simulink model "sampleModel1919"  (R2023a)
settings: Solver=VariableStepAuto  StartTime=0.0  StopTime=10.0  RelTol=1e-3
libraries: hdlsllib x6, simulink x1
settings Model: Creator=user1  LastModifiedBy=user1

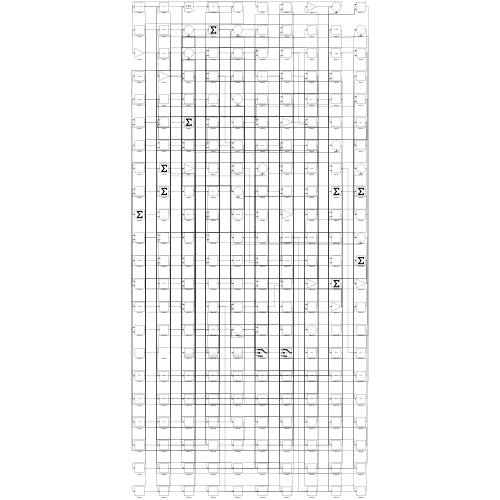
[thumbnail: Simulink's stored preview of the top-level diagram]
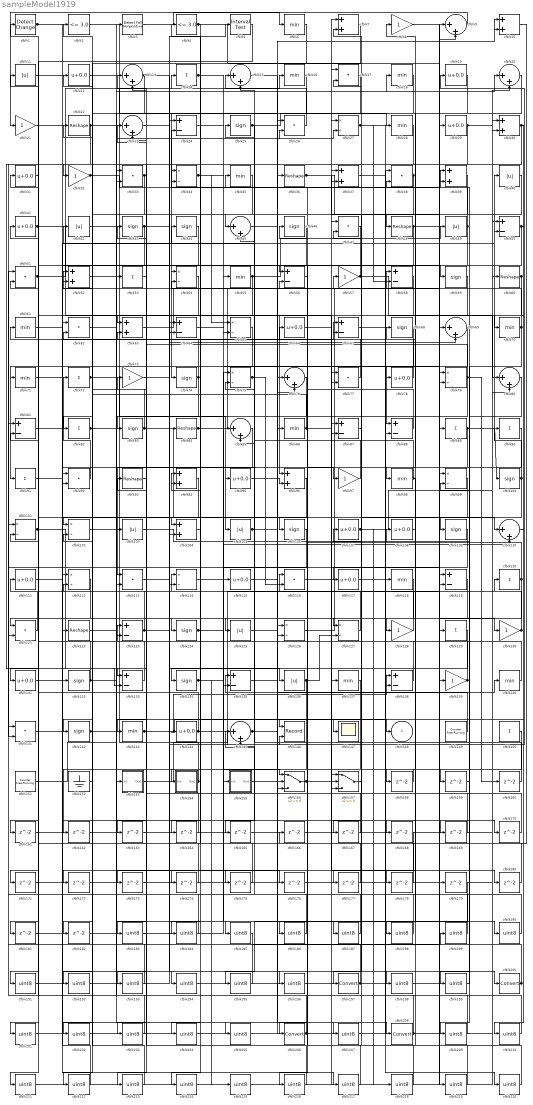
== system sampleModel1919 ==
  cfblk1 : simulink/Logic and Bit Operations/Detect Change  vinit=0  OutDataTypeStr=boolean
      settings: LibrarySourceBlock=|
      | hdlsllib/Logic and Bit
      | Operations/Detect
      | Change
  cfblk{7,10,30,37,39,52,63,94,96,104} (10 alike) : Sum
  cfblk{25,43..44,46,59,68,74,83,100,106,109,124,132,134,142} (15 alike) : Signum
  cfblk{27,34,54,65,75,79,99,101..102,112,114,126..127} (13 alike) : Product  Inputs=*/  RndMeth=Zero  SaturateOnIntegerOverflow=on
  cfblk{11,40,42,49,103,105,125,136} (8 alike) : Abs  SaturateOnIntegerOverflow=off
  cfblk{12,19,29,31,41,66,78,95,107..108,111,115,117,131,144} (15 alike) : Bias  Bias=0.0  SaturateOnIntegerOverflow=off
  cfblk{9,13,15,20,23,45,69,76,80,85,110,145} (12 alike) : Sum  Inputs=|++
  cfblk{17,26,33,38,47,51,62,77,92,113,116,121,141} (13 alike) : DotProduct  OutDataTypeStr=Inherit: Inherit via internal rule
  cfblk{6,16,18,28,35,55,61,70..71,86,98,118,137,140,143} (15 alike) : MinMax
  cfblk{24,50,56,58,64,67,81,87..88,119,123,133,135,138} (14 alike) : Sum  Inputs=+-
  cfblk{14,53,72,82,89..91,120,129} (9 alike) : Sum  Inputs=+
  cfblk{22,36,48,60,84,93,122} (7 alike) : Reshape
  cfblk{8,21,32,57,73,97,128,130,139} (9 alike) : Gain
  cfblk146 : Record  FileSettingsInternal="{\"entries\":[{\"content\":{\"excelSettings\":{\"content\":{},\"type\":\"Streamout.ExcelSettings\"}},\"type\":\"Streamout.FileSettingStorage\",\"uuid\":\"\"}],\"packageUris\":[\"http:\\/\\/schema.mathworks.com\\/mf0\\/streamout_blocks\\/R2020a\"],\"version\":\"1.0\"}"  Layout=[1 1]  SignalsInternal="{\"entries\":[{\"content\":{\"signals\":[{\"content\":{\"blockPath\":[],\"dimensions\":[1],\"domain\":\"\",\"lineColor\":\"#a2142f\",\"plots\":[1],\"port\":1,\"signalID\":5132,\"signalName\":\"XY Graph:1\"},\"type\":\"RecordBlkView.Signal\",\"uuid\":\"\"},{\"content\":{\"blockPath\":[],\"dimensions\":[1],\"domain\":\"\",\"lineColor\":\"#139fff\",\"plots\":[1],\"port\":2,\"signalID\":5135,\"signalName\":\"XY Graph:2\"},\"type\":\"RecordBlkView.Signal\",\"uuid\":\"\"}]},\"type\":\"RecordBlkView.InputSignals\",\"uuid\":\"\"}],\"packageUris\":[\"http:\\/\\/schema.mathworks.com\\/mf0\\/streamout_blocks\\/R2020a\"],\"version\":\"1.0\"}"  VisualizationBindings="{\"xyplotplugin\":{\"info\":[{\"series\":[{\"bindingParametersList\":[{\"parameter\":\"X-Axis\",\"signalID\":5132,\"signalName\":\"XY Graph:1\"},{\"parameter\":\"Y-Axis\",\"signalID\":5135,\"signalName\":\"XY Graph:2\"}],\"seriesID\":65422}],\"subplotID\":1}]}}"  CompatibilityTag=XY  st=-1
  cfblk147 : Scope
  cfblk149 : hdlsllib/Sources/Counter Free-Running  NumBits=16  tsamp=-1
  cfblk150 : Constant  SampleTime=-1
  cfblk151 : hdlsllib/Sources/Counter Free-Running  NumBits=16  tsamp=-1
  cfblk152 : Ground
  cfblk153 : Subsystem
      settings: LibrarySourceBlock=|
      | hdlsllib/Ports &
      | Subsystems/Subsystem
  cfblk154 : Subsystem
      settings: LibrarySourceBlock=|
      | hdlsllib/Ports &
      | Subsystems/Subsystem
  cfblk155 : Subsystem
      settings: LibrarySourceBlock=|
      | hdlsllib/Ports &
      | Subsystems/Subsystem
  cfblk156 : Switch  SaturateOnIntegerOverflow=off  InputSameDT=off
  cfblk157 : Switch  SaturateOnIntegerOverflow=off  InputSameDT=off
  cfblk{158..182} (25 alike) : Delay  SampleTime=1
  cfblk{183..196,198..199,201..205,207,209..220} (34 alike) : DataTypeConversion  OutDataTypeStr=uint8  SaturateOnIntegerOverflow=off  RndMeth=Floor
  cfblk{197,200,206,208} (4 alike) : DataTypeConversion  SaturateOnIntegerOverflow=off  RndMeth=Floor
  cfblk2 : hdlsllib/Logic and Bit Operations/Compare To Constant  relop=<=  const=3.0  OutDataTypeStr=boolean
  cfblk3 : hdlsllib/Logic and Bit Operations/Detect Fall Nonpositive  vinit=0  OutDataTypeStr=boolean
  cfblk4 : hdlsllib/Logic and Bit Operations/Compare To Constant  relop=<=  const=3.0  OutDataTypeStr=boolean
  cfblk5 : hdlsllib/Logic and Bit Operations/Interval Test  IntervalClosedRight=on  uplimit=0.5  IntervalClosedLeft=on  lowlimit=-0.5  OutDataTypeStr=boolean
  cfblk148 : Outport  VectorParamsAs1DForOutWhenUnconnected=off
  wires:
  cfblk83/1 -> cfblk109/1, cfblk52/1, cfblk196/1
  cfblk126/1 -> cfblk39/1
  cfblk92/1 -> cfblk72/1
  cfblk26/1 -> cfblk15/1
  cfblk131/1 -> cfblk132/1
  cfblk88/1 -> cfblk35/1
  cfblk100/1 -> cfblk40/1, cfblk128/1
  cfblk121/1 -> cfblk111/1
  cfblk6/1 -> cfblk82/1
  cfblk63/1 -> cfblk57/1
  cfblk15/1 -> cfblk126/1
  cfblk154/1(Out1) -> cfblk14/1, cfblk13/1
  cfblk123/1 -> cfblk31/1, cfblk136/1
  cfblk51/1 -> cfblk16/1, cfblk135/2
  cfblk16/1 -> cfblk74/1
  cfblk66/1 -> cfblk7/1
  cfblk119/1 -> cfblk124/1
  cfblk143/1 -> cfblk138/1, cfblk13/2, cfblk5/1, cfblk146/2
  cfblk65/1 -> cfblk91/1
  cfblk9/1 -> cfblk21/1
  cfblk86/1 -> cfblk83/1, cfblk52/2, cfblk180/1
  cfblk57/1 -> cfblk54/1, cfblk80/1
  cfblk89/1 -> cfblk100/1, cfblk127/1
  cfblk7/1 -> cfblk104/1
  cfblk134/1 -> cfblk110/2, cfblk215/1
  cfblk116/1 -> cfblk29/1
  cfblk85/1 -> cfblk113/1
  cfblk78/1 -> cfblk15/2
  cfblk69/1 -> cfblk133/1
  cfblk39/1 -> cfblk117/1
  cfblk96/1 -> cfblk121/1
  cfblk5/1 -> cfblk133/2
  cfblk17/1 -> cfblk134/1
  cfblk77/1 -> cfblk61/1
  cfblk13/1 -> cfblk32/1, cfblk85/1
  cfblk25/1 -> cfblk28/1, cfblk95/1
  cfblk50/1 -> cfblk144/1, cfblk181/1
  cfblk29/1 -> cfblk20/2, cfblk191/1
  cfblk144/1 -> cfblk19/1, cfblk101/2
  cfblk128/1 -> cfblk114/1
  cfblk127/1 -> cfblk12/1
  cfblk136/1 -> cfblk127/2, cfblk162/1
  cfblk33/1 -> cfblk163/1, cfblk202/1
  cfblk53/1 -> cfblk143/1
  cfblk19/1 -> cfblk98/1
  cfblk4/1 -> cfblk139/1, cfblk204/1
  cfblk156/1 -> cfblk116/1, cfblk10/1
  cfblk59/1 -> cfblk96/1
  cfblk22/1 -> cfblk147/1, cfblk141/2
  cfblk107/1 -> cfblk30/1, cfblk218/1
  cfblk32/1 -> cfblk39/2, cfblk20/1
  cfblk105/1 -> cfblk10/2, cfblk165/1
  cfblk55/1 -> cfblk49/1, cfblk65/2
  cfblk130/1 -> cfblk120/1, cfblk85/2
  cfblk12/1 -> cfblk55/1
  cfblk138/1 -> cfblk11/1
  cfblk23/1 -> cfblk84/1
  cfblk36/1 -> cfblk119/1, cfblk48/1
  cfblk151/1 -> cfblk53/1
  cfblk115/1 -> cfblk26/1
  cfblk42/1 -> cfblk26/2
  cfblk35/1 -> cfblk102/1
  cfblk103/1 -> cfblk108/1
  cfblk152/1 -> cfblk2/1
  cfblk70/1 -> cfblk54/2, cfblk199/1
  cfblk60/1 -> cfblk145/2, cfblk167/1
  cfblk46/1 -> cfblk113/2
  cfblk90/1 -> cfblk206/1
  cfblk113/1 -> cfblk69/2
  cfblk38/1 -> cfblk45/1, cfblk156/3
  cfblk75/1 -> cfblk25/1, cfblk116/2
  cfblk3/1 -> cfblk6/1
  cfblk49/1 -> cfblk24/2, cfblk213/1
  cfblk44/1 -> cfblk63/1
  cfblk157/1 -> cfblk107/1
  cfblk27/1 -> cfblk118/1, cfblk58/2
  cfblk84/1 -> cfblk9/2, cfblk4/1
  cfblk21/1 -> cfblk97/1
  cfblk24/1 -> cfblk156/1
  cfblk14/1 -> cfblk119/2, cfblk77/2
  cfblk82/1 -> cfblk104/2, cfblk182/1
  cfblk67/1 -> cfblk138/2
  cfblk132/1 -> cfblk41/1, cfblk205/1
  cfblk118/1 -> cfblk131/1
  cfblk30/1 -> cfblk70/1, cfblk92/2
  cfblk11/1 -> cfblk56/1
  cfblk142/1 -> cfblk18/1, cfblk175/1
  cfblk133/1 -> cfblk123/1
  cfblk79/1 -> cfblk23/2, cfblk156/2, cfblk160/1
  cfblk106/1 -> cfblk121/2
  cfblk135/1 -> cfblk86/1
  cfblk48/1 -> cfblk130/1, cfblk154/1(In1), cfblk184/1
  cfblk153/1(Out1) -> cfblk89/1
  cfblk99/1 -> cfblk197/1
  cfblk74/1 -> cfblk43/1, cfblk114/2
  cfblk41/1 -> cfblk87/2, cfblk59/1
  cfblk43/1 -> cfblk142/1, cfblk176/1
  cfblk61/1 -> cfblk50/2
  cfblk37/1 -> cfblk200/1
  cfblk54/1 -> cfblk71/1
  cfblk95/1 -> cfblk96/2
  cfblk120/1 -> cfblk66/1, cfblk186/1, cfblk201/1
  cfblk155/1(Out1) -> cfblk140/1
  cfblk2/1 -> cfblk36/1
  cfblk98/1 -> cfblk34/1, cfblk44/1, cfblk158/1
  cfblk149/1 -> cfblk135/1
  cfblk97/1 -> cfblk42/1
  cfblk101/1 -> cfblk153/1(In1), cfblk56/2
  cfblk71/1 -> cfblk67/1
  cfblk122/1 -> cfblk27/2
  cfblk102/1 -> cfblk110/1
  cfblk140/1 -> cfblk68/1
  cfblk72/1 -> cfblk105/1, cfblk192/1
  cfblk139/1 -> cfblk58/1, cfblk94/2, cfblk75/2
  cfblk68/1 -> cfblk88/1
  cfblk124/1 -> cfblk75/1, cfblk94/1
  cfblk81/1 -> cfblk208/1
  cfblk145/1 -> cfblk168/1, cfblk169/1
  cfblk56/1 -> cfblk146/1
  cfblk1/1 -> cfblk122/1, cfblk106/1
  cfblk45/1 -> cfblk79/2
  cfblk34/1 -> cfblk155/1(In1), cfblk65/1
  cfblk20/1 -> cfblk33/2
  cfblk114/1 -> cfblk148/1
  cfblk52/1 -> cfblk103/1
  cfblk40/1 -> cfblk125/1
  cfblk87/1 -> cfblk17/2
  cfblk158/1 -> cfblk157/2
  cfblk80/1 -> cfblk159/1
  cfblk160/1 -> cfblk45/2
  cfblk31/1 -> cfblk161/1
  cfblk161/1 -> cfblk79/1
  cfblk162/1 -> cfblk126/2
  cfblk163/1 -> cfblk69/1
  cfblk104/1 -> cfblk164/1
  cfblk164/1 -> cfblk24/1
  cfblk165/1 -> cfblk50/1
  cfblk10/1 -> cfblk166/1
  cfblk166/1 -> cfblk9/1
  cfblk167/1 -> cfblk157/1
  cfblk169/1 -> cfblk123/2
  cfblk91/1 -> cfblk170/1
  cfblk170/1 -> cfblk87/1
  cfblk58/1 -> cfblk171/1
  cfblk171/1 -> cfblk38/1
  cfblk94/1 -> cfblk172/1
  cfblk172/1 -> cfblk88/2
  cfblk28/1 -> cfblk173/1
  cfblk173/1 -> cfblk27/1
  cfblk18/1 -> cfblk174/1
  cfblk174/1 -> cfblk23/1
  cfblk175/1 -> cfblk34/2
  cfblk176/1 -> cfblk30/2
  cfblk109/1 -> cfblk177/1
  cfblk177/1 -> cfblk1/1
  cfblk108/1 -> cfblk178/1
  cfblk178/1 -> cfblk17/1
  cfblk180/1 -> cfblk102/2
  cfblk182/1 -> cfblk3/1
  cfblk93/1 -> cfblk183/1
  cfblk183/1 -> cfblk115/1
  cfblk184/1 -> cfblk93/1
  cfblk73/1 -> cfblk185/1
  cfblk186/1 -> cfblk73/1
  cfblk62/1 -> cfblk187/1
  cfblk187/1 -> cfblk145/1
  cfblk150/1 -> cfblk188/1
  cfblk188/1 -> cfblk62/1
  cfblk185/1 -> cfblk189/1
  cfblk189/1 -> cfblk62/2
  cfblk64/1 -> cfblk190/1
  cfblk190/1 -> cfblk141/1
  cfblk191/1 -> cfblk64/1
  cfblk192/1 -> cfblk64/2
  cfblk137/1 -> cfblk193/1
  cfblk193/1 -> cfblk22/1
  cfblk111/1 -> cfblk194/1
  cfblk194/1 -> cfblk137/1
  cfblk179/1 -> cfblk195/1
  cfblk195/1 -> cfblk51/2
  cfblk196/1 -> cfblk179/1
  cfblk197/1 -> cfblk101/1, cfblk77/1
  cfblk181/1 -> cfblk198/1
  cfblk198/1 -> cfblk99/1
  cfblk199/1 -> cfblk99/2
  cfblk200/1 -> cfblk92/1, cfblk7/2
  cfblk201/1 -> cfblk37/1
  cfblk202/1 -> cfblk37/2
  cfblk76/1 -> cfblk203/1
  cfblk203/1 -> cfblk51/1
  cfblk204/1 -> cfblk76/1
  cfblk205/1 -> cfblk76/2
  cfblk206/1 -> cfblk78/1, cfblk33/1
  cfblk125/1 -> cfblk207/1
  cfblk207/1 -> cfblk90/1
  cfblk208/1 -> cfblk38/2, cfblk80/2, cfblk67/2
  cfblk159/1 -> cfblk209/1
  cfblk209/1 -> cfblk81/1
  cfblk110/1 -> cfblk210/1
  cfblk210/1 -> cfblk81/2
  cfblk112/1 -> cfblk211/1
  cfblk211/1 -> cfblk60/1
  cfblk168/1 -> cfblk212/1
  cfblk212/1 -> cfblk112/1
  cfblk213/1 -> cfblk112/2
  cfblk129/1 -> cfblk214/1
  cfblk214/1 -> cfblk157/3
  cfblk215/1 -> cfblk129/1
  cfblk47/1 -> cfblk216/1
  cfblk216/1 -> cfblk63/2
  cfblk141/1 -> cfblk217/1
  cfblk217/1 -> cfblk47/1
  cfblk218/1 -> cfblk47/2
  cfblk8/1 -> cfblk219/1
  cfblk219/1 -> cfblk46/1
  cfblk117/1 -> cfblk220/1
  cfblk220/1 -> cfblk8/1

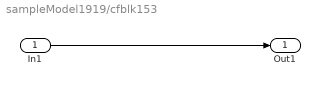
== system sampleModel1919/cfblk153 ==
  In1 : Inport
  Out1 : Outport
  wires:
  In1/1 -> Out1/1

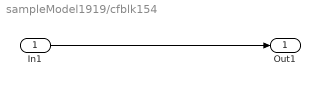
== system sampleModel1919/cfblk154 ==
  In1 : Inport
  Out1 : Outport
  wires:
  In1/1 -> Out1/1

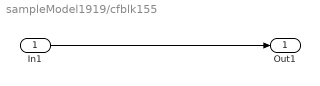
== system sampleModel1919/cfblk155 ==
  In1 : Inport
  Out1 : Outport
  wires:
  In1/1 -> Out1/1
